simulink model "MINI_Simscape_IK"  (R2021a)
settings: Solver=VariableStepAuto  StartTime=0.0  StopTime=10  FixedStep=0.01  MaxStep=0.01  RelTol=1e-3
model workspace: external: MATLAB File .\MINI_DataFile.m (data not in the file)
undefined symbols (not defined in the file or in its folder): smiData, X, Y, Z
libraries: sm_lib x368, nesl_utility x17
(part 7 of 7)

== system MINI_Simscape_IK/Left Arm/L_arm_03_1_RIGID/hands_L_1_RIGID/SPL_2b2_8_RIGID ==
  ReferenceFrame : sm_lib/Frames and Transforms/Reference Frame
  Solid : sm_lib/Body Elements/File Solid  ExtGeomFileName=SPL-2b2.STEP  UnitType=FromFile  ExtGeomFileUnits=m  StepReaderType=HEX  ExportConvexHullGeometry=off  InertiaType=Custom  Mass=smiData.Solid(7).mass  MassUnits=kg  CenterOfMass=smiData.Solid(7).CoM  CenterOfMassUnits=mm  MomentsOfInertia=smiData.Solid(7).MoI  MomentsOfInertiaUnits=kg*mm^2  ProductsOfInertia=smiData.Solid(7).PoI  ProductsOfInertiaUnits=kg*mm^2  BasedOnType=DensityFromFile  Density=1000  DensityUnits=kg/m^3  DoExposeReferenceFrame=on  SerializedFrames=<Frames/>  GraphicType=FromGeometry  MarkerShape=Sphere  MarkerSize=10  GraphicVisPropType=SimpleVisualProperties  GraphicDiffuseColor=smiData.Solid(7).color  GraphicSpecularColor=[0.5 0.5 0.5 1.0]  GraphicAmbientColor=[0.15 0.15 0.15 1.0]  GraphicEmissiveColor=[0.0 0.0 0.0 1.0]  GraphicShininess=75  GraphicOpacity=smiData.Solid(7).opacity
  F : PMIOPort  Side=Left
  connections:
  Solid/RConn1 -- ReferenceFrame/RConn1 -- F/RConn1

== system MINI_Simscape_IK/Left Arm/L_arm_03_1_RIGID/hands_L_1_RIGID/SPL_2b2_9_RIGID ==
  ReferenceFrame : sm_lib/Frames and Transforms/Reference Frame
  Solid : sm_lib/Body Elements/File Solid  ExtGeomFileName=SPL-2b2.STEP  UnitType=FromFile  ExtGeomFileUnits=m  StepReaderType=HEX  ExportConvexHullGeometry=off  InertiaType=Custom  Mass=smiData.Solid(7).mass  MassUnits=kg  CenterOfMass=smiData.Solid(7).CoM  CenterOfMassUnits=mm  MomentsOfInertia=smiData.Solid(7).MoI  MomentsOfInertiaUnits=kg*mm^2  ProductsOfInertia=smiData.Solid(7).PoI  ProductsOfInertiaUnits=kg*mm^2  BasedOnType=DensityFromFile  Density=1000  DensityUnits=kg/m^3  DoExposeReferenceFrame=on  SerializedFrames=<Frames/>  GraphicType=FromGeometry  MarkerShape=Sphere  MarkerSize=10  GraphicVisPropType=SimpleVisualProperties  GraphicDiffuseColor=smiData.Solid(7).color  GraphicSpecularColor=[0.5 0.5 0.5 1.0]  GraphicAmbientColor=[0.15 0.15 0.15 1.0]  GraphicEmissiveColor=[0.0 0.0 0.0 1.0]  GraphicShininess=75  GraphicOpacity=smiData.Solid(7).opacity
  F : PMIOPort  Side=Left
  connections:
  Solid/RConn1 -- ReferenceFrame/RConn1 -- F/RConn1

== system MINI_Simscape_IK/Left Arm/L_arm_03_1_RIGID/hands_L_1_RIGID/SPU_5_1_RIGID ==
  ReferenceFrame : sm_lib/Frames and Transforms/Reference Frame
  Solid : sm_lib/Body Elements/File Solid  ExtGeomFileName=SPU-5.STEP  UnitType=FromFile  ExtGeomFileUnits=m  StepReaderType=HEX  ExportConvexHullGeometry=off  InertiaType=Custom  Mass=smiData.Solid(8).mass  MassUnits=kg  CenterOfMass=smiData.Solid(8).CoM  CenterOfMassUnits=mm  MomentsOfInertia=smiData.Solid(8).MoI  MomentsOfInertiaUnits=kg*mm^2  ProductsOfInertia=smiData.Solid(8).PoI  ProductsOfInertiaUnits=kg*mm^2  BasedOnType=DensityFromFile  Density=1000  DensityUnits=kg/m^3  DoExposeReferenceFrame=on  SerializedFrames=<Frames/>  GraphicType=FromGeometry  MarkerShape=Sphere  MarkerSize=10  GraphicVisPropType=SimpleVisualProperties  GraphicDiffuseColor=smiData.Solid(8).color  GraphicSpecularColor=[0.5 0.5 0.5 1.0]  GraphicAmbientColor=[0.15 0.15 0.15 1.0]  GraphicEmissiveColor=[0.0 0.0 0.0 1.0]  GraphicShininess=75  GraphicOpacity=smiData.Solid(8).opacity
  F : PMIOPort  Side=Left
  connections:
  Solid/RConn1 -- ReferenceFrame/RConn1 -- F/RConn1

== system MINI_Simscape_IK/Right Arm/R_arm_03_1_RIGID/hands_R_1_RIGID/SP0_5_1_RIGID ==
  ReferenceFrame : sm_lib/Frames and Transforms/Reference Frame
  Solid : sm_lib/Body Elements/File Solid  ExtGeomFileName=SP0-5.STEP  UnitType=FromFile  ExtGeomFileUnits=m  StepReaderType=HEX  ExportConvexHullGeometry=off  InertiaType=Custom  Mass=smiData.Solid(2).mass  MassUnits=kg  CenterOfMass=smiData.Solid(2).CoM  CenterOfMassUnits=mm  MomentsOfInertia=smiData.Solid(2).MoI  MomentsOfInertiaUnits=kg*mm^2  ProductsOfInertia=smiData.Solid(2).PoI  ProductsOfInertiaUnits=kg*mm^2  BasedOnType=DensityFromFile  Density=1000  DensityUnits=kg/m^3  DoExposeReferenceFrame=on  SerializedFrames=<Frames/>  GraphicType=FromGeometry  MarkerShape=Sphere  MarkerSize=10  GraphicVisPropType=SimpleVisualProperties  GraphicDiffuseColor=smiData.Solid(2).color  GraphicSpecularColor=[0.5 0.5 0.5 1.0]  GraphicAmbientColor=[0.15 0.15 0.15 1.0]  GraphicEmissiveColor=[0.0 0.0 0.0 1.0]  GraphicShininess=75  GraphicOpacity=smiData.Solid(2).opacity
  F : PMIOPort  Side=Left
  connections:
  Solid/RConn1 -- ReferenceFrame/RConn1 -- F/RConn1

== system MINI_Simscape_IK/Right Arm/R_arm_03_1_RIGID/hands_R_1_RIGID/SPD_1_RIGID ==
  ReferenceFrame : sm_lib/Frames and Transforms/Reference Frame
  Solid : sm_lib/Body Elements/File Solid  ExtGeomFileName=SPD_3b3.STEP  UnitType=FromFile  ExtGeomFileUnits=m  StepReaderType=HEX  ExportConvexHullGeometry=off  InertiaType=Custom  Mass=smiData.Solid(5).mass  MassUnits=kg  CenterOfMass=smiData.Solid(5).CoM  CenterOfMassUnits=mm  MomentsOfInertia=smiData.Solid(5).MoI  MomentsOfInertiaUnits=kg*mm^2  ProductsOfInertia=smiData.Solid(5).PoI  ProductsOfInertiaUnits=kg*mm^2  BasedOnType=DensityFromFile  Density=1000  DensityUnits=kg/m^3  DoExposeReferenceFrame=on  SerializedFrames=<Frames/>  GraphicType=FromGeometry  MarkerShape=Sphere  MarkerSize=10  GraphicVisPropType=SimpleVisualProperties  GraphicDiffuseColor=smiData.Solid(5).color  GraphicSpecularColor=[0.5 0.5 0.5 1.0]  GraphicAmbientColor=[0.15 0.15 0.15 1.0]  GraphicEmissiveColor=[0.0 0.0 0.0 1.0]  GraphicShininess=75  GraphicOpacity=smiData.Solid(5).opacity
  F : PMIOPort  Side=Left
  connections:
  Solid/RConn1 -- ReferenceFrame/RConn1 -- F/RConn1

== system MINI_Simscape_IK/Right Arm/R_arm_03_1_RIGID/hands_R_1_RIGID/SPD_2_RIGID ==
  ReferenceFrame : sm_lib/Frames and Transforms/Reference Frame
  Solid : sm_lib/Body Elements/File Solid  ExtGeomFileName=SPD_3b5.STEP  UnitType=FromFile  ExtGeomFileUnits=m  StepReaderType=HEX  ExportConvexHullGeometry=off  InertiaType=Custom  Mass=smiData.Solid(4).mass  MassUnits=kg  CenterOfMass=smiData.Solid(4).CoM  CenterOfMassUnits=mm  MomentsOfInertia=smiData.Solid(4).MoI  MomentsOfInertiaUnits=kg*mm^2  ProductsOfInertia=smiData.Solid(4).PoI  ProductsOfInertiaUnits=kg*mm^2  BasedOnType=DensityFromFile  Density=1000  DensityUnits=kg/m^3  DoExposeReferenceFrame=on  SerializedFrames=<Frames/>  GraphicType=FromGeometry  MarkerShape=Sphere  MarkerSize=10  GraphicVisPropType=SimpleVisualProperties  GraphicDiffuseColor=smiData.Solid(4).color  GraphicSpecularColor=[0.5 0.5 0.5 1.0]  GraphicAmbientColor=[0.15 0.15 0.15 1.0]  GraphicEmissiveColor=[0.0 0.0 0.0 1.0]  GraphicShininess=75  GraphicOpacity=smiData.Solid(4).opacity
  F : PMIOPort  Side=Left
  connections:
  Solid/RConn1 -- ReferenceFrame/RConn1 -- F/RConn1

== system MINI_Simscape_IK/Right Arm/R_arm_03_1_RIGID/hands_R_1_RIGID/SPD_4_RIGID ==
  ReferenceFrame : sm_lib/Frames and Transforms/Reference Frame
  Solid : sm_lib/Body Elements/File Solid  ExtGeomFileName=SPD_4b5.STEP  UnitType=FromFile  ExtGeomFileUnits=m  StepReaderType=HEX  ExportConvexHullGeometry=off  InertiaType=Custom  Mass=smiData.Solid(6).mass  MassUnits=kg  CenterOfMass=smiData.Solid(6).CoM  CenterOfMassUnits=mm  MomentsOfInertia=smiData.Solid(6).MoI  MomentsOfInertiaUnits=kg*mm^2  ProductsOfInertia=smiData.Solid(6).PoI  ProductsOfInertiaUnits=kg*mm^2  BasedOnType=DensityFromFile  Density=1000  DensityUnits=kg/m^3  DoExposeReferenceFrame=on  SerializedFrames=<Frames/>  GraphicType=FromGeometry  MarkerShape=Sphere  MarkerSize=10  GraphicVisPropType=SimpleVisualProperties  GraphicDiffuseColor=smiData.Solid(6).color  GraphicSpecularColor=[0.5 0.5 0.5 1.0]  GraphicAmbientColor=[0.15 0.15 0.15 1.0]  GraphicEmissiveColor=[0.0 0.0 0.0 1.0]  GraphicShininess=75  GraphicOpacity=smiData.Solid(6).opacity
  F : PMIOPort  Side=Left
  connections:
  Solid/RConn1 -- ReferenceFrame/RConn1 -- F/RConn1

== system MINI_Simscape_IK/Right Arm/R_arm_03_1_RIGID/hands_R_1_RIGID/SPD_9_RIGID ==
  ReferenceFrame : sm_lib/Frames and Transforms/Reference Frame
  Solid : sm_lib/Body Elements/File Solid  ExtGeomFileName=SPD_3b5.STEP  UnitType=FromFile  ExtGeomFileUnits=m  StepReaderType=HEX  ExportConvexHullGeometry=off  InertiaType=Custom  Mass=smiData.Solid(4).mass  MassUnits=kg  CenterOfMass=smiData.Solid(4).CoM  CenterOfMassUnits=mm  MomentsOfInertia=smiData.Solid(4).MoI  MomentsOfInertiaUnits=kg*mm^2  ProductsOfInertia=smiData.Solid(4).PoI  ProductsOfInertiaUnits=kg*mm^2  BasedOnType=DensityFromFile  Density=1000  DensityUnits=kg/m^3  DoExposeReferenceFrame=on  SerializedFrames=<Frames/>  GraphicType=FromGeometry  MarkerShape=Sphere  MarkerSize=10  GraphicVisPropType=SimpleVisualProperties  GraphicDiffuseColor=smiData.Solid(4).color  GraphicSpecularColor=[0.5 0.5 0.5 1.0]  GraphicAmbientColor=[0.15 0.15 0.15 1.0]  GraphicEmissiveColor=[0.0 0.0 0.0 1.0]  GraphicShininess=75  GraphicOpacity=smiData.Solid(4).opacity
  F : PMIOPort  Side=Left
  connections:
  Solid/RConn1 -- ReferenceFrame/RConn1 -- F/RConn1

== system MINI_Simscape_IK/Right Arm/R_arm_03_1_RIGID/hands_R_1_RIGID/SPL_2b2_10_RIGID ==
  ReferenceFrame : sm_lib/Frames and Transforms/Reference Frame
  Solid : sm_lib/Body Elements/File Solid  ExtGeomFileName=SPL-2b2.STEP  UnitType=FromFile  ExtGeomFileUnits=m  StepReaderType=HEX  ExportConvexHullGeometry=off  InertiaType=Custom  Mass=smiData.Solid(7).mass  MassUnits=kg  CenterOfMass=smiData.Solid(7).CoM  CenterOfMassUnits=mm  MomentsOfInertia=smiData.Solid(7).MoI  MomentsOfInertiaUnits=kg*mm^2  ProductsOfInertia=smiData.Solid(7).PoI  ProductsOfInertiaUnits=kg*mm^2  BasedOnType=DensityFromFile  Density=1000  DensityUnits=kg/m^3  DoExposeReferenceFrame=on  SerializedFrames=<Frames/>  GraphicType=FromGeometry  MarkerShape=Sphere  MarkerSize=10  GraphicVisPropType=SimpleVisualProperties  GraphicDiffuseColor=smiData.Solid(7).color  GraphicSpecularColor=[0.5 0.5 0.5 1.0]  GraphicAmbientColor=[0.15 0.15 0.15 1.0]  GraphicEmissiveColor=[0.0 0.0 0.0 1.0]  GraphicShininess=75  GraphicOpacity=smiData.Solid(7).opacity
  F : PMIOPort  Side=Left
  connections:
  Solid/RConn1 -- ReferenceFrame/RConn1 -- F/RConn1

== system MINI_Simscape_IK/Right Arm/R_arm_03_1_RIGID/hands_R_1_RIGID/SPL_2b2_11_RIGID ==
  ReferenceFrame : sm_lib/Frames and Transforms/Reference Frame
  Solid : sm_lib/Body Elements/File Solid  ExtGeomFileName=SPL-2b2.STEP  UnitType=FromFile  ExtGeomFileUnits=m  StepReaderType=HEX  ExportConvexHullGeometry=off  InertiaType=Custom  Mass=smiData.Solid(7).mass  MassUnits=kg  CenterOfMass=smiData.Solid(7).CoM  CenterOfMassUnits=mm  MomentsOfInertia=smiData.Solid(7).MoI  MomentsOfInertiaUnits=kg*mm^2  ProductsOfInertia=smiData.Solid(7).PoI  ProductsOfInertiaUnits=kg*mm^2  BasedOnType=DensityFromFile  Density=1000  DensityUnits=kg/m^3  DoExposeReferenceFrame=on  SerializedFrames=<Frames/>  GraphicType=FromGeometry  MarkerShape=Sphere  MarkerSize=10  GraphicVisPropType=SimpleVisualProperties  GraphicDiffuseColor=smiData.Solid(7).color  GraphicSpecularColor=[0.5 0.5 0.5 1.0]  GraphicAmbientColor=[0.15 0.15 0.15 1.0]  GraphicEmissiveColor=[0.0 0.0 0.0 1.0]  GraphicShininess=75  GraphicOpacity=smiData.Solid(7).opacity
  F : PMIOPort  Side=Left
  connections:
  Solid/RConn1 -- ReferenceFrame/RConn1 -- F/RConn1

== system MINI_Simscape_IK/Right Arm/R_arm_03_1_RIGID/hands_R_1_RIGID/SPL_2b2_1_RIGID ==
  ReferenceFrame : sm_lib/Frames and Transforms/Reference Frame
  Solid : sm_lib/Body Elements/File Solid  ExtGeomFileName=SPL-2b2.STEP  UnitType=FromFile  ExtGeomFileUnits=m  StepReaderType=HEX  ExportConvexHullGeometry=off  InertiaType=Custom  Mass=smiData.Solid(7).mass  MassUnits=kg  CenterOfMass=smiData.Solid(7).CoM  CenterOfMassUnits=mm  MomentsOfInertia=smiData.Solid(7).MoI  MomentsOfInertiaUnits=kg*mm^2  ProductsOfInertia=smiData.Solid(7).PoI  ProductsOfInertiaUnits=kg*mm^2  BasedOnType=DensityFromFile  Density=1000  DensityUnits=kg/m^3  DoExposeReferenceFrame=on  SerializedFrames=<Frames/>  GraphicType=FromGeometry  MarkerShape=Sphere  MarkerSize=10  GraphicVisPropType=SimpleVisualProperties  GraphicDiffuseColor=smiData.Solid(7).color  GraphicSpecularColor=[0.5 0.5 0.5 1.0]  GraphicAmbientColor=[0.15 0.15 0.15 1.0]  GraphicEmissiveColor=[0.0 0.0 0.0 1.0]  GraphicShininess=75  GraphicOpacity=smiData.Solid(7).opacity
  F : PMIOPort  Side=Left
  connections:
  Solid/RConn1 -- ReferenceFrame/RConn1 -- F/RConn1

== system MINI_Simscape_IK/Right Arm/R_arm_03_1_RIGID/hands_R_1_RIGID/SPL_2b2_2_RIGID ==
  ReferenceFrame : sm_lib/Frames and Transforms/Reference Frame
  Solid : sm_lib/Body Elements/File Solid  ExtGeomFileName=SPL-2b2.STEP  UnitType=FromFile  ExtGeomFileUnits=m  StepReaderType=HEX  ExportConvexHullGeometry=off  InertiaType=Custom  Mass=smiData.Solid(7).mass  MassUnits=kg  CenterOfMass=smiData.Solid(7).CoM  CenterOfMassUnits=mm  MomentsOfInertia=smiData.Solid(7).MoI  MomentsOfInertiaUnits=kg*mm^2  ProductsOfInertia=smiData.Solid(7).PoI  ProductsOfInertiaUnits=kg*mm^2  BasedOnType=DensityFromFile  Density=1000  DensityUnits=kg/m^3  DoExposeReferenceFrame=on  SerializedFrames=<Frames/>  GraphicType=FromGeometry  MarkerShape=Sphere  MarkerSize=10  GraphicVisPropType=SimpleVisualProperties  GraphicDiffuseColor=smiData.Solid(7).color  GraphicSpecularColor=[0.5 0.5 0.5 1.0]  GraphicAmbientColor=[0.15 0.15 0.15 1.0]  GraphicEmissiveColor=[0.0 0.0 0.0 1.0]  GraphicShininess=75  GraphicOpacity=smiData.Solid(7).opacity
  F : PMIOPort  Side=Left
  connections:
  Solid/RConn1 -- ReferenceFrame/RConn1 -- F/RConn1

== system MINI_Simscape_IK/Right Arm/R_arm_03_1_RIGID/hands_R_1_RIGID/SPL_2b2_7_RIGID ==
  ReferenceFrame : sm_lib/Frames and Transforms/Reference Frame
  Solid : sm_lib/Body Elements/File Solid  ExtGeomFileName=SPL-2b2.STEP  UnitType=FromFile  ExtGeomFileUnits=m  StepReaderType=HEX  ExportConvexHullGeometry=off  InertiaType=Custom  Mass=smiData.Solid(7).mass  MassUnits=kg  CenterOfMass=smiData.Solid(7).CoM  CenterOfMassUnits=mm  MomentsOfInertia=smiData.Solid(7).MoI  MomentsOfInertiaUnits=kg*mm^2  ProductsOfInertia=smiData.Solid(7).PoI  ProductsOfInertiaUnits=kg*mm^2  BasedOnType=DensityFromFile  Density=1000  DensityUnits=kg/m^3  DoExposeReferenceFrame=on  SerializedFrames=<Frames/>  GraphicType=FromGeometry  MarkerShape=Sphere  MarkerSize=10  GraphicVisPropType=SimpleVisualProperties  GraphicDiffuseColor=smiData.Solid(7).color  GraphicSpecularColor=[0.5 0.5 0.5 1.0]  GraphicAmbientColor=[0.15 0.15 0.15 1.0]  GraphicEmissiveColor=[0.0 0.0 0.0 1.0]  GraphicShininess=75  GraphicOpacity=smiData.Solid(7).opacity
  F : PMIOPort  Side=Left
  connections:
  Solid/RConn1 -- ReferenceFrame/RConn1 -- F/RConn1

== system MINI_Simscape_IK/Right Arm/R_arm_03_1_RIGID/hands_R_1_RIGID/SPL_2b2_8_RIGID ==
  ReferenceFrame : sm_lib/Frames and Transforms/Reference Frame
  Solid : sm_lib/Body Elements/File Solid  ExtGeomFileName=SPL-2b2.STEP  UnitType=FromFile  ExtGeomFileUnits=m  StepReaderType=HEX  ExportConvexHullGeometry=off  InertiaType=Custom  Mass=smiData.Solid(7).mass  MassUnits=kg  CenterOfMass=smiData.Solid(7).CoM  CenterOfMassUnits=mm  MomentsOfInertia=smiData.Solid(7).MoI  MomentsOfInertiaUnits=kg*mm^2  ProductsOfInertia=smiData.Solid(7).PoI  ProductsOfInertiaUnits=kg*mm^2  BasedOnType=DensityFromFile  Density=1000  DensityUnits=kg/m^3  DoExposeReferenceFrame=on  SerializedFrames=<Frames/>  GraphicType=FromGeometry  MarkerShape=Sphere  MarkerSize=10  GraphicVisPropType=SimpleVisualProperties  GraphicDiffuseColor=smiData.Solid(7).color  GraphicSpecularColor=[0.5 0.5 0.5 1.0]  GraphicAmbientColor=[0.15 0.15 0.15 1.0]  GraphicEmissiveColor=[0.0 0.0 0.0 1.0]  GraphicShininess=75  GraphicOpacity=smiData.Solid(7).opacity
  F : PMIOPort  Side=Left
  connections:
  Solid/RConn1 -- ReferenceFrame/RConn1 -- F/RConn1

== system MINI_Simscape_IK/Right Arm/R_arm_03_1_RIGID/hands_R_1_RIGID/SPL_2b2_9_RIGID ==
  ReferenceFrame : sm_lib/Frames and Transforms/Reference Frame
  Solid : sm_lib/Body Elements/File Solid  ExtGeomFileName=SPL-2b2.STEP  UnitType=FromFile  ExtGeomFileUnits=m  StepReaderType=HEX  ExportConvexHullGeometry=off  InertiaType=Custom  Mass=smiData.Solid(7).mass  MassUnits=kg  CenterOfMass=smiData.Solid(7).CoM  CenterOfMassUnits=mm  MomentsOfInertia=smiData.Solid(7).MoI  MomentsOfInertiaUnits=kg*mm^2  ProductsOfInertia=smiData.Solid(7).PoI  ProductsOfInertiaUnits=kg*mm^2  BasedOnType=DensityFromFile  Density=1000  DensityUnits=kg/m^3  DoExposeReferenceFrame=on  SerializedFrames=<Frames/>  GraphicType=FromGeometry  MarkerShape=Sphere  MarkerSize=10  GraphicVisPropType=SimpleVisualProperties  GraphicDiffuseColor=smiData.Solid(7).color  GraphicSpecularColor=[0.5 0.5 0.5 1.0]  GraphicAmbientColor=[0.15 0.15 0.15 1.0]  GraphicEmissiveColor=[0.0 0.0 0.0 1.0]  GraphicShininess=75  GraphicOpacity=smiData.Solid(7).opacity
  F : PMIOPort  Side=Left
  connections:
  Solid/RConn1 -- ReferenceFrame/RConn1 -- F/RConn1

== system MINI_Simscape_IK/Right Arm/R_arm_03_1_RIGID/hands_R_1_RIGID/SPU_5_1_RIGID ==
  ReferenceFrame : sm_lib/Frames and Transforms/Reference Frame
  Solid : sm_lib/Body Elements/File Solid  ExtGeomFileName=SPU-5.STEP  UnitType=FromFile  ExtGeomFileUnits=m  StepReaderType=HEX  ExportConvexHullGeometry=off  InertiaType=Custom  Mass=smiData.Solid(8).mass  MassUnits=kg  CenterOfMass=smiData.Solid(8).CoM  CenterOfMassUnits=mm  MomentsOfInertia=smiData.Solid(8).MoI  MomentsOfInertiaUnits=kg*mm^2  ProductsOfInertia=smiData.Solid(8).PoI  ProductsOfInertiaUnits=kg*mm^2  BasedOnType=DensityFromFile  Density=1000  DensityUnits=kg/m^3  DoExposeReferenceFrame=on  SerializedFrames=<Frames/>  GraphicType=FromGeometry  MarkerShape=Sphere  MarkerSize=10  GraphicVisPropType=SimpleVisualProperties  GraphicDiffuseColor=smiData.Solid(8).color  GraphicSpecularColor=[0.5 0.5 0.5 1.0]  GraphicAmbientColor=[0.15 0.15 0.15 1.0]  GraphicEmissiveColor=[0.0 0.0 0.0 1.0]  GraphicShininess=75  GraphicOpacity=smiData.Solid(8).opacity
  F : PMIOPort  Side=Left
  connections:
  Solid/RConn1 -- ReferenceFrame/RConn1 -- F/RConn1

== matlab function MINI_Simscape_IK/MATLAB Function1 ==
  data: x_RH_in input; th1 output; y_RH_in input; z_RH_in input; th3 output; th5 output
% ECE 598 JK Fall 2020 University of Illinois at Urbana-Champaign
% ROBOTIS MINI Right Hand Inverse Kinematics
% 09/07/2020 by Kevin Gim (kggim2@illinois.edu)

function [th1,th3,th5] = IK_RH(x_RH_in, y_RH_in, z_RH_in)

L_sh = 39; % Origin to arm roll joint
L_a1 = 18; % Shoulder bracket horizontal distance
L_a2 = 12; % Shoulder bracket vertical distance
L_a3 = 45; % Upper arm length
L_a4 = 72; % Lower arm length

% Position of Right hand in Initial Pose (all the right arm motor angle == 0)
% x_0 = 0;
% y_0 = -174;
% z_0 = -12;
x_0 = 0;
y_0 = 0;
z_0 = 0;


th1 = 0;
th3 = 0;
th5 = 0;


% Right Arm
x_RH = x_0 + x_RH_in;
y_RH = y_0 + y_RH_in;
z_RH = z_0 + z_RH_in;
x_RH0 = x_RH;
y_RH0 = y_RH + (L_sh + L_a1);
z_RH0 = z_RH;

th1 = -atan(x_RH0/(z_RH0+0.00001))

% Range of XL320 motor -150 to 150 deg
if (th1 > 2.618)
    th1 = 2.618;
elseif (th1 < -2.618)
    th1 = -2.618;
else
    th1 = th1;
end

R1_RH = sqrt((x_RH0 - L_a2*sin(th1))^2 + y_RH0^2 + (z_RH0 + L_a2*cos(th1))^2);

if (R1_RH > 117)
    R1_RH = 117
else
    R1_RH = R1_RH;
end

alpha_RH = acos((L_a3^2 + L_a4^2 -R1_RH^2)/(2*L_a3*L_a4));

% Elbow Joint angle
th5 = -pi + alpha_RH
R2_RH = sqrt((x_RH0 - L_a2*sin(th1))^2 + (z_RH0 + L_a2*cos(th1))^2);

% Shoulder Joint angle
if (z_RH > 0)
th3 = pi/2 + (atan(y_RH0/R2_RH) + acos((L_a3^2 + R1_RH^2 - L_a4^2)/(2*L_a3*R1_RH)));
else
th3 = -pi/2 + (-atan(y_RH0/R2_RH) + acos((L_a3^2 + R1_RH^2 - L_a4^2)/(2*L_a3*R1_RH)));
end

== matlab function MINI_Simscape_IK/MATLAB Function2 ==
  data: x_LH_in input; th2 output; th4 output; th6 output; y_LH_in input; z_LH_in input
% ECE 598 JK Fall 2020 University of Illinois at Urbana-Champaign
% ROBOTIS MINI Left Hand Inverse Kinematics
% 09/07/2020 by Kevin Gim (kggim2@illinois.edu)


function [th2,th4,th6] = IK_LH(x_LH_in, y_LH_in, z_LH_in)

L_sh = 39; % Origin to arm roll joint
L_a1 = 18; % Shoulder bracket horizontal distance
L_a2 = 12; % Shoulder bracket vertical distance
L_a3 = 45; % Upper arm length
L_a4 = 72; % Lower arm length

% Position of Left hand in Initial Pose (all the left arm motor angle == 0)
% x_0 = 0;
% y_0 = 174;
% z_0 = -12;
x_0 = 0;
y_0 = 0;
z_0 = 0;

th2 = 0;
th4 = 0;
th6 = 0;

% Left Arm
x_LH = x_0 + x_LH_in;
y_LH = y_0 + y_LH_in;
z_LH = z_0 + z_LH_in;

x_LH0 = x_LH;
y_LH0 = y_LH - (L_sh + L_a1);
z_LH0 = z_LH;

th2 = atan(x_LH0/(z_LH0+0.00001));

% Range of XL320 motor -150 to 150 deg
if (th2 > 2.618)
    th2 = 2.618;
elseif (th2 < -2.618)
    th2 = -2.618;
else
    th2 = th2;
end

R1_LH = sqrt((x_LH0 - L_a2*sin(th2))^2 + y_LH0^2 + (z_LH0+L_a2*cos(th2))^2);

if (R1_LH > 117)
    R1_LH = 117;
else
    R1_LH = R1_LH;
end

alpha_LH = acos((L_a3^2 + L_a4^2 -R1_LH^2)/(2*L_a3*L_a4));

% Elbow Joint angle 
th6 = pi - alpha_LH;

R2_LH = sqrt((x_LH0 - L_a2*sin(th2))^2 + (z_LH0 + L_a2*cos(th2))^2);

% Shoulder Joint angle
if (z_LH0 > 0)
    th4 = -((atan(R2_LH/y_LH0) + acos((L_a3^2 + R1_LH^2 - L_a4^2)/(2*L_a3*R1_LH))));
else
    th4 = -(-pi/2 + (atan(y_LH0/R2_LH) + acos((L_a3^2 + R1_LH^2 - L_a4^2)/(2*L_a3*R1_LH))));
end

== matlab function MINI_Simscape_IK/MATLAB Function ==
  data: x_LF_in input; th8 output; y_LF_in input; z_LF_in input; roll_LF input; pitch_LF input; th10 output; th12 output; th14 output; th16 output
% ECE 598 JK Fall 2020 University of Illinois at Urbana-Champaign
% ROBOTIS MINI Left Foot Inverse Kinematics
% 09/07/2020 by Kevin Gim (kggim2@illinois.edu)

function [th8, th10, th12, th14, th16] = IK_LF(x_LF_in, y_LF_in, z_LF_in, roll_LF, pitch_LF)

%Left foot
% Controllable position x, y, z, roll, pitch

L_by = 24; % Origin to pelvis vertical length
L_bz = 72; % Pelvis horizontal length
L_bx = 15; % Shoulder joint axis to Leg center (On Sagittal Plane)
L_l1 = 6;  % Pelvis Roll axis to pitch axis
L_l2 = 45; % Thigh Length
L_l3 = 42; % Shank Length
L_l4 = 31;  % Ankle Length
L_f = 9; % Foot horizontal length

% x_0 = 15; y_0 = 24; z_0 = -196;
x_0 = 0; y_0 = 0; z_0 = 0;
x_LF = x_0 + x_LF_in;
y_LF = y_0 + y_LF_in;
z_LF = z_0 + z_LF_in;


R0LF = RX(roll_LF) * RY(pitch_LF);
T0LF = R0LF + TXYZ(x_LF, y_LF, z_LF) - eye(4);
T016 = T0LF * RY(-(pi)/2) *RZ((pi)) * TXYZ(-L_l4,0,0);
TLF0_16 = inv(TXYZ(L_bx,L_by,-L_bz)*RY((pi)/2))*T016;
pos_LF = TLF0_16(1:3,4);

th8 = atan(pos_LF(2)/pos_LF(1))
R1_LF = sqrt((pos_LF(1)-L_l1*cos(th8))^2 + (pos_LF(2)-L_l1*sin(th8))^2 + pos_LF(3)^2);
alpha_LF = acos((L_l2^2 + L_l3^2 -R1_LF^2)/(2*L_l2*L_l3));

th12 = -pi+alpha_LF
R2_LF = sqrt((pos_LF(1)-L_l1*cos(th8))^2 + (pos_LF(2)-L_l1*sin(th8))^2);

th10 = (atan(pos_LF(3)/R2_LF) + acos((L_l2^2 + R1_LF^2 - L_l3^2)/(2*L_l2*R1_LF)));


T_LF0_12 = [ cos(th10 + th12)*cos(th8), -sin(th10 + th12)*cos(th8),  sin(th8), cos(th8)*(L_l1 + L_l2*cos(th10));
    cos(th10 + th12)*sin(th8), -sin(th10 + th12)*sin(th8), -cos(th8), sin(th8)*(L_l1 + L_l2*cos(th10));
    sin(th10 + th12),           cos(th10 + th12),         0,                   L_l2*sin(th10);
    0,                          0,         0,                                1]

T_12_16 = inv(T_LF0_12)*TLF0_16;
th14 = -acos(-T_12_16(2,3));
th16 = asin(-T_12_16(3,1));

== matlab function MINI_Simscape_IK/MATLAB Function3 ==
  data: x_RF_in input; th7 output; y_RF_in input; z_RF_in input; roll_RF input; pitch_RF input; th9 output; th11 output; th13 output; th15 output
% ECE 598 JK Fall 2020 University of Illinois at Urbana-Champaign
% ROBOTIS MINI Right Foot Inverse Kinematics
% 09/07/2020 by Kevin Gim (kggim2@illinois.edu)

function [th7,th9, th11, th13, th15] = IK_RF(x_RF_in, y_RF_in, z_RF_in, roll_RF, pitch_RF)

% Right foot
% Controllable position x, y, z, roll, pitch

L_by = 24; % Origin to pelvis vertical length
L_bz = 72; % Pelvis horizontal length
L_bx = 15; % Shoulder joint axis to Leg center (On Sagittal Plane)
L_l1 = 6;  % Pelvis Roll axis to pitch axis
L_l2 = 45; % Thigh Length
L_l3 = 42; % Shank Length
L_l4 = 31;  % Ankle Length
L_f = 9; % Foot horizontal length

% x_0 = 15; y_0 = -24; z_0 = -196;
x_0 = 0; y_0 = 0; z_0 = 0;

x_RF = x_0 + x_RF_in;
y_RF = y_0 + y_RF_in;
z_RF = z_0 + z_RF_in;

R0RF = RX(roll_RF) * RY(pitch_RF);
T0RF = R0RF + TXYZ(x_RF, y_RF, z_RF) - eye(4);
T015 = T0RF * RY(-(pi)/2) * RZ((pi)) * TXYZ(-L_l4,0,0);
TRF0_15 = inv(TXYZ(L_bx,-L_by,-L_bz)*RY((pi)/2))*T015;

pos_RF = TRF0_15(1:3,4);
th7 = atan(pos_RF(2)/pos_RF(1))
R1_RF = sqrt((pos_RF(1)-L_l1*cos(th7))^2 + (pos_RF(2)-L_l1*sin(th7))^2 + pos_RF(3)^2);
alpha_RF = acos((L_l2^2 + L_l3^2 -R1_RF^2)/(2*L_l2*L_l3));
th11 = pi-alpha_RF
R2_RF = sqrt((pos_RF(1)-L_l1*cos(th7))^2 + (pos_RF(2)-L_l1*sin(th7))^2);

th9 = -((atan(pos_RF(3)/R2_RF) + acos((L_l2^2 + R1_RF^2 - L_l3^2)/(2*L_l2*R1_RF))));

T_RF0_11 = [ cos(th9 + th11)*cos(th7), -sin(th9 + th11)*cos(th7), -sin(th7), cos(th7)*(L_l1 + L_l2*cos(th9));
    cos(th9 + th11)*sin(th7), -sin(th9 + th11)*sin(th7),  cos(th7), sin(th7)*(L_l1 + L_l2*cos(th9));
    -sin(th9 + th11),          -cos(th9 + th11),         0,                  -L_l2*sin(th9);
    0,                         0,         0,                               1];

T_11_15 = inv(T_RF0_11)*TRF0_15;
th13 = asin(T_11_15(1,3));
th15 = -asin(-T_11_15(3,1));
